simulink model "laserGameSimul"  (R2023a)
settings: Solver=VariableStepAuto  StartTime=0.0  StopTime=Tsim  RelTol=1e-3
values from neighbouring files (symbols this model uses):
  omega1 = 2*pi*f1    (= 534070.75111)    [laserGame.m]
  omega2 = 2*pi*f2    (= 565486.677646)    [laserGame.m]
  omega3 = 2*pi*f3    (= 596902.604182)    [laserGame.m]
  omega4 = 2*pi*f4    (= 628318.530718)    [laserGame.m]
  omega5 = 2*pi*f5    (= 722566.310326)    [laserGame.m]
  omega6 = 2*pi*f6    (= 753982.236862)    [laserGame.m]
  Te = T/M    (= 0.00446428571429)    [ScriptDFT.m]    (also in laserGame.m = 3.125e-06)
settings Model: Creator=iben-brahim  LastModifiedBy=doumbouya

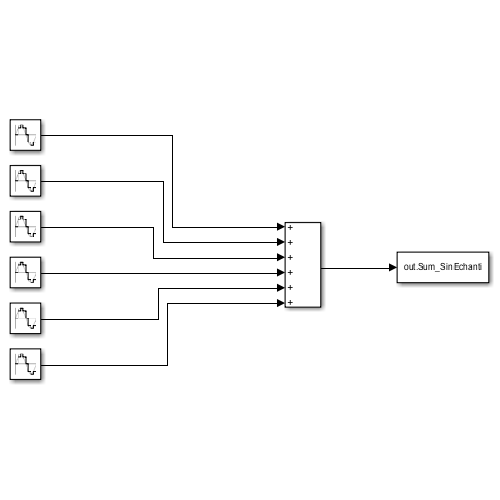
[thumbnail: Simulink's stored preview of the top-level diagram]
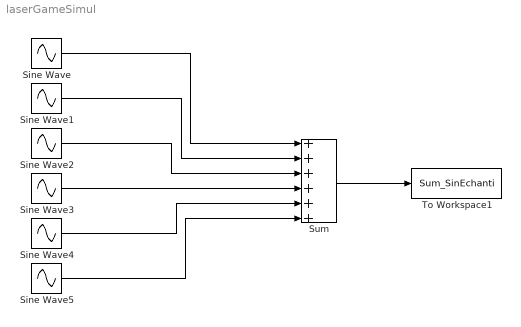
== system laserGameSimul ==
  Sine Wave : Sin  Frequency=omega1  SampleTime=Te
  Sine Wave1 : Sin  Frequency=omega2  SampleTime=Te
  Sine Wave2 : Sin  Frequency=omega3  SampleTime=Te
  Sine Wave3 : Sin  Frequency=omega4  SampleTime=Te
  Sine Wave4 : Sin  Frequency=omega5  SampleTime=Te
  Sine Wave5 : Sin  Frequency=omega6  SampleTime=Te
  Sum : Sum  Inputs=6
  To Workspace1 : ToWorkspace  VariableName=Sum_SinEchanti  SaveFormat=Timeseries  SampleTime=-1
  wires:
  Sine Wave/1 -> Sum/1
  Sine Wave1/1 -> Sum/2
  Sine Wave2/1 -> Sum/3
  Sine Wave3/1 -> Sum/4
  Sine Wave4/1 -> Sum/5
  Sine Wave5/1 -> Sum/6
  Sum/1 -> To Workspace1/1
